simulink model "tanqueSimulink"  (R2021b)
settings: Solver=VariableStepAuto  StartTime=0.0  StopTime=1000  RelTol=1e-3
values from neighbouring files (symbols this model uses):
  a = 2.1382    [tanque.m]
  A = 389.16    [tanque.m]
  g = 9.8    [tanque.m]
settings Model: Creator=cesar  LastModifiedBy=cesar
settings SolverCC: AlgebraicLoopSolver=TrustRegion
settings DebuggingCC: SFMachineParentedDataDiag=warning

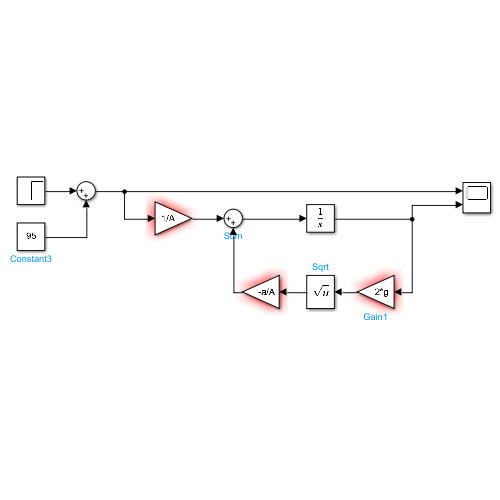
[thumbnail: Simulink's stored preview of the top-level diagram]
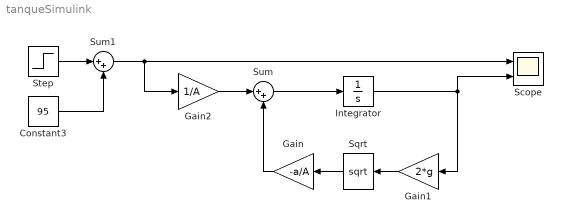
== system tanqueSimulink ==
  Constant3 : Constant  Value=95
  Gain : Gain  Gain=-a/A
  Gain1 : Gain  Gain=2*g
  Gain2 : Gain  Gain=1/A
  Integrator : Integrator  InitialCondition=1.006
  Scope : Scope  NumInputPorts=2
  Sqrt : Sqrt  SaturateOnIntegerOverflow=on
  Step : Step  Time=200  After=30  SampleTime=0
  Sum : Sum  Inputs=|++
  Sum1 : Sum  Inputs=|++
  wires:
  Constant3/1 -> Sum1/2
  Gain2/1 -> Sum/1
  Gain1/1 -> Sqrt/1
  Gain/1 -> Sum/2
  Sum/1 -> Integrator/1
  Integrator/1 -> Scope/2, Gain1/1
  Step/1 -> Sum1/1
  Sum1/1 -> Gain2/1, Scope/1
  Sqrt/1 -> Gain/1
